simulink model "Rocket"  (R2025b)
settings: Solver=VariableStepAuto  StartTime=0.0  StopTime=3  MaxStep=0.01  RelTol=1e-3  AbsTol=1e-6
values from neighbouring files (symbols this model uses):
  thrust_N = [0, 311.629, 351.768, 349.074, 346.175, 341.229, 336.857, 333.748,                 326.960, 319.679, 312.533, 300.790, 292.787, 283.766, 274.578,                 264.915, 254.273, 241.755, 229.020, 216.238, 187.776, 109.940,                 56.459,  24.476,  10.977,   3.450,   0.000]    [thrust_data.m]
  time_thrust = [0, 0.028, 0.087, 0.147, 0.206, 0.266, 0.325, 0.384,                 0.444, 0.503, 0.563, 0.622, 0.681, 0.741, 0.800,                 0.859, 0.919, 0.978, 1.037, 1.097, 1.156, 1.216,                 1.275, 1.334, 1.394, 1.454, 1.515]    [thrust_data.m]
undefined symbols (not defined in the file or in its folder): A_ref
libraries: aerolib6dof2 x1, slpidlib x1
settings Model: Creator=kang  LastModifiedBy=kang

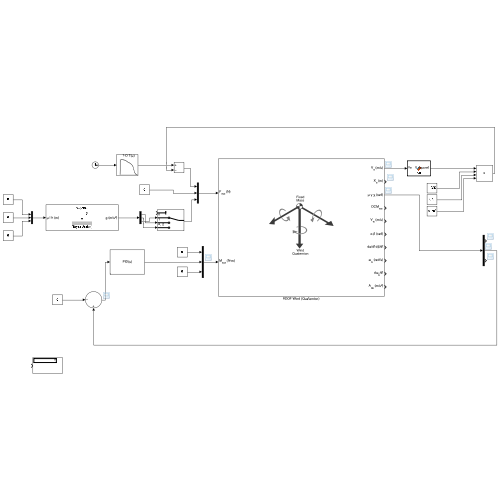
[thumbnail: Simulink's stored preview of the top-level diagram]
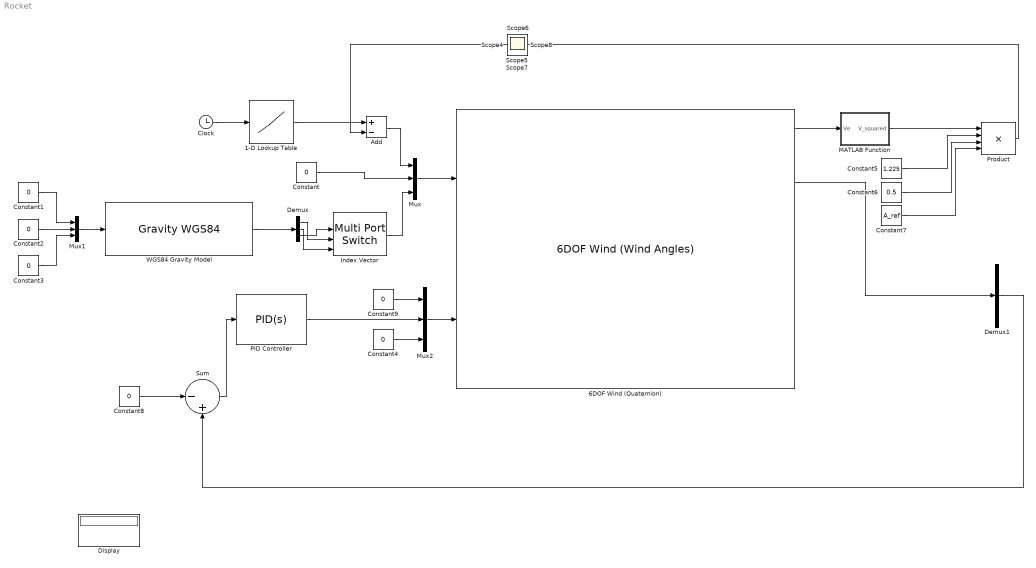
== system Rocket ==
  1-D Lookup Table : Lookup_n-D  NumberOfTableDimensions=1  LookupTableObject=thrust_data  BreakpointsForDimension1=time_thrust  Table=thrust_N  InternalRulePriority=Speed  RndMeth=Simplest
  6DOF Wind (Quaternion) : aerolib6dof2/6DOF Wind (Wind Angles)  units=Metric (MKS)  mtype=Fixed  rep=Quaternion  xme_0=[0 0 0]  Vm_0=[0.001 0 0]  wind_0=[0 0 0]  pm_0=[0.01 0.5 0.5]  mass_0=total_mass  mass_e=0.5  mass_f=2.0  inertia=eye(3)  inertia_e=eye(3)  inertia_f=2*eye(3)  vre_flag=on  abi_flag=off  xme_statename=''  Vm_statename=''  alpha_statename=''  beta_statename=''  wind_statename=''  quat_statename=''  pm_statename=''  mass_statename=''
      settings: LibrarySourceBlock=aerolib6dof2/6DOF Wind (Quaternion)
  Add : Sum  Inputs=+-
  Clock : Clock
  Constant{,1..4,8..9} (7 alike) : Constant  Value=0
  Constant5 : Constant  Value=1.225
  Constant6 : Constant  Value=0.5
  Constant7 : Constant  Value=A_ref
  Demux : Demux  Outputs=3
  Demux1 : Demux  Outputs=3
  Display : Display
  Index Vector : MultiPortSwitch  DataPortOrder=Zero-based contiguous  zeroidx=on  SaturateOnIntegerOverflow=off  InputSameDT=off
  MATLAB Function : MATLAB Function  TreatAsAtomicUnit=on
  Mux : Mux  Inputs=3
  Mux1 : Mux  Inputs=3
  Mux2 : Mux  Inputs=3
  PID Controller : slpidlib/PID Controller  Controller=PID  Form=Parallel  TimeDomain=Continuous-time  UseExternalTs=off  SampleTime=-1  IntegratorMethod=Forward Euler  FilterMethod=Forward Euler  ControllerParametersSource=internal  P=50000  I=0  UseKiTs=off  D=500  UseExternalDerivativeSource=off  N=100  UseFilter=on  TunerSelectOption=Transfer Function Based (PID Tuner App)  InitialConditionSource=internal  InitialConditionForIntegrator=0  InitialConditionForFilter=0  DifferentiatorICPrevScaledInput=0  ExternalReset=none  TrackingMode=off  Kt=1  LimitOutput=off  SatLimitsSource=internal  UpperSaturationLimit=inf  LowerSaturationLimit=-inf  LinearizeAsGain=on  AntiWindupMode=none  Kb=1  LimitIntegrator=off  UpperIntegratorSaturationLimit=inf  LowerIntegratorSaturationLimit=-inf  POutMin=[]  POutMax=[]  IOutMin=[]  IOutMax=[]  DOutMin=[]  DOutMax=[]  NOutMin=[]  NOutMax=[]  SumOutMin=[]  SumOutMax=[]  SaturationOutMin=[]  SaturationOutMax=[]  PParamMin=[]  PParamMax=[]  IParamMin=[]  IParamMax=[]  DParamMin=[]  DParamMax=[]  NParamMin=[]  NParamMax=[]  KbParamMin=[]  KbParamMax=[]  KtParamMin=[]  KtParamMax=[]  KbOutMin=[]  KbOutMax=[]  KtOutMin=[]  KtOutMax=[]  IntegratorOutMin=[]  IntegratorOutMax=[]  FilterOutMin=[]  FilterOutMax=[]  SumI1OutMin=[]  SumI1OutMax=[]  SumI2OutMin=[]  SumI2OutMax=[]  SumI3OutMin=[]  SumI3OutMax=[]  SumI4OutMin=[]  SumI4OutMax=[]  SumDOutMin=[]  SumDOutMax=[]  DifferentiatorOutMin=[]  DifferentiatorOutMax=[]  FilterDiffOutCoefMin=[]  FilterDiffOutCoefMax=[]  ReciprocalOutMin=[]  ReciprocalOutMax=[]  SumDenOutMin=[]  SumDenOutMax=[]  SumNumOutMin=[]  SumNumOutMax=[]  DivideOutMin=[]  DivideOutMax=[]  UdiffTsProdOutMin=[]  UdiffTsProdOutMax=[]  NTsProdOutMin=[]  NTsProdOutMax=[]  UintegralTsProdOutMin=[]  UintegralTsProdOutMax=[]  UngainTsProdOutMin=[]  UngainTsProdOutMax=[]  ClampingZeroOutDataTypeStr=Inherit: Inherit via back propagation  ClampingZeroOutMin=[]  ClampingZeroOutMax=[]  FilterDenConstantOutDataTypeStr=Inherit: Inherit via back propagation  FilterDenConstantOutMin=[]  FilterDenConstantOutMax=[]  PCopyOutDataTypeStr=Inherit: Inherit via back propagation  PCopyOutMin=[]  PCopyOutMax=[]  NCopyOutDataTypeStr=Inherit: Inherit via back propagation  NCopyOutMin=[]  NCopyOutMax=[]  IntegratorContinuousStateAttributes=''  IntegratorStateMustResolveToSignalObject=off  IntegratorRTWStateStorageClass=Auto  FilterContinuousStateAttributes=''  FilterStateMustResolveToSignalObject=off  FilterRTWStateStorageClass=Auto  ParallelPVariant=InternalParameters  IdealPVariant=Disabled  IVariant=InternalParameters  DVariant=InternalParameters  IntegratorVariant=Continuous  SatVariant=Disabled  AWVariant=Passthrough  PCopyVariant=Disabled  TRVariant=Disabled  FdbkBlocksVariant=Forward  IdealPFdbkVariant=Disabled  SatFdbkVariant=Disabled  DerivativeFilterVariant=ContFilter  NVariant=InternalParameters  NCopyVariant=Disabled  FilterICVariant=InternalICsFilter  IntegratorICVariant=InternalICs  ExternalResetVariant=Disabled  TRSumVariant=Passthrough  SumFdbkVariant=Disabled  SumVariant=Sum_PID  TsampFilterVariant=InternalTs  TsampNgainVariant=Passthrough  TsampIntegralVariant=Disabled_SignalSpec  ExternalSaturationOutDataTypeStr=Inherit: Same as second input  DerivativeSourceVariant=ErrorSignal  PreIntVariant=InternalPreInt
  Product : Product  Inputs=4
  Sum : Sum  Inputs=|-+
  "WGS84 Gravity Model  " : GravityWGS84
  Scope{,1..8} (9 alike) : Scope
      Scope settings: ActiveDisplayYMinimum=-1  ActiveDisplayYMaximum=1
      Scope1 settings: ActiveDisplayYMinimum=-1  ActiveDisplayYMaximum=1
      Scope2 settings: ActiveDisplayYMinimum=-1.2908711646844364  ActiveDisplayYMaximum=3.6340886333980409  DataLoggingVariableName=ScopeData2
      Scope3 settings: ActiveDisplayYMinimum=-1  ActiveDisplayYMaximum=1  DataLoggingVariableName=ScopeData3
      Scope4 settings: ActiveDisplayYMinimum=-1  ActiveDisplayYMaximum=1  DataLoggingVariableName=ScopeData4
      Scope5 settings: ActiveDisplayYMinimum=-3.9268560113327884  ActiveDisplayYMaximum=3.9269742315015268  DataLoggingVariableName=ScopeData5
      Scope6 settings: ActiveDisplayYMinimum=-1  ActiveDisplayYMaximum=1  DataLoggingVariableName=ScopeData6
      Scope7 settings: ActiveDisplayYMinimum=-1  ActiveDisplayYMaximum=1  DataLoggingVariableName=ScopeData7
      Scope8 settings: ActiveDisplayYMinimum=-1  ActiveDisplayYMaximum=1  DataLoggingVariableName=ScopeData8
  wires:
  Constant/1 -> Mux/2
  Mux/1 -> 6DOF Wind (Quaternion)/1
  Clock/1 -> 1-D Lookup Table/1
  Constant2/1 -> Mux1/2
  Constant1/1 -> Mux1/1
  Constant3/1 -> Mux1/3
  Mux1/1 -> "WGS84 Gravity Model  "/1
  Mux2/1 -> 6DOF Wind (Quaternion)/2
  Index Vector/1 -> Mux/3
  "WGS84 Gravity Model  "/1 -> Demux/1
  Demux/3 -> Index Vector/2
  Demux/1 -> Index Vector/3
  Demux/2 -> Index Vector/4
  Constant5/1 -> Product/2
  Constant6/1 -> Product/3
  Constant7/1 -> Product/4
  MATLAB Function/1(V_squared) -> Product/1
  1-D Lookup Table/1 -> Add/1
  Product/1 -> Add/2
  Add/1 -> Mux/1
  6DOF Wind (Quaternion)/1 -> MATLAB Function/1(Ve)
  6DOF Wind (Quaternion)/3 -> Demux1/1
  Demux1/2 -> Sum/2
  Constant8/1 -> Sum/1
  Sum/1 -> PID Controller/1
  Constant9/1 -> Mux2/1
  Constant4/1 -> Mux2/3
  PID Controller/1 -> Mux2/2

== matlab function Rocket/MATLAB Function ==
  data: Ve input; V_squared output
function V_squared = fcn(Ve)
    V_squared = Ve(1)^2 + Ve(2)^2 + Ve(3)^2;
end
